simulink model "Tractor_Model"  (R2022b)
settings: Solver=daessc  StartTime=0.0  StopTime=80  FixedStep=1  MaxStep=.01  RelTol=1
libraries: nesl_utility x12, fl_lib x6, sdl_lib x5, simulink x2
settings Model: Creator=david  LastModifiedBy=david
settings SolverCC: ZeroCrossAlgorithm=Adaptive
settings SimscapeCC: SimscapeLogType=all

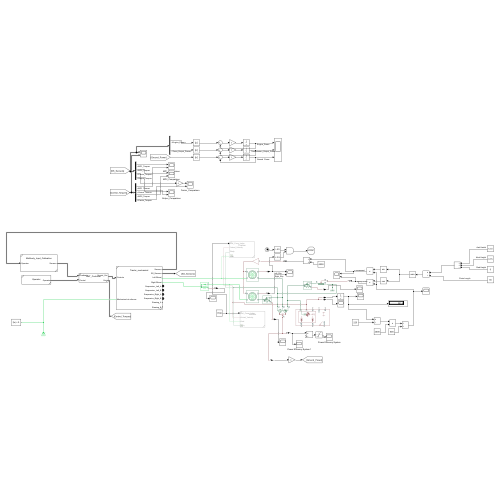
[thumbnail: Simulink's stored preview of the top-level diagram]
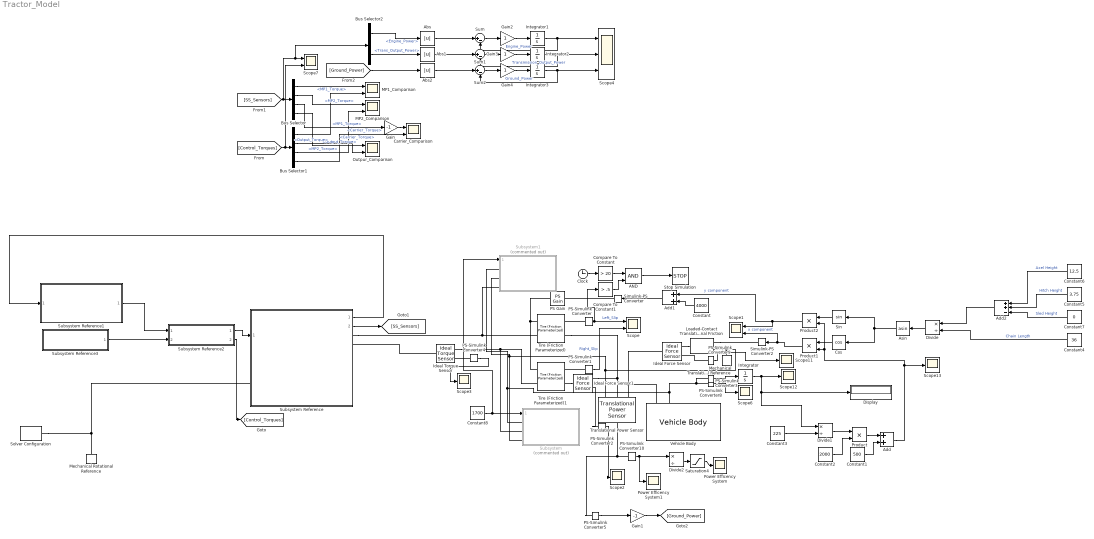
== system Tractor_Model ==
  AND : Logic  IconShape=distinctive  AllPortsSameDT=off  OutDataTypeStr=boolean
  Abs : Abs  SaturateOnIntegerOverflow=off
  Abs1 : Abs  SaturateOnIntegerOverflow=off
  Abs2 : Abs  SaturateOnIntegerOverflow=off
  Add : Sum
  Add1 : Sum
  Add2 : Sum  Inputs=++-
  Asin : Trigonometry  Operator=asin
  Bus Selector : BusSelector  OutputSignals=Trans.MP1_Torque,Trans.MP2_Torque,Trans.Carrier_Torque,Trans.Output_Torque
  Bus Selector1 : BusSelector  OutputSignals=MP1_Torque,Output_Torque,MP2_Torque,Carrier_Torque
  Bus Selector2 : BusSelector  OutputSignals=Engine_Power,Trans_Output_Power
  Carrier_Comparison : Scope  NumInputPorts=2
  Clock : Clock
  Compare To Constant : simulink/Logic and Bit Operations/Compare To Constant  relop=>  const=20  OutDataTypeStr=boolean
  Compare To Constant1 : simulink/Logic and Bit Operations/Compare To Constant  relop=>  const=.5  OutDataTypeStr=boolean
  Constant : Constant  Value=4000
  Constant1 : Constant  Value=500
  Constant2 : Constant  Value=2000
  Constant3 : Constant  Value=225
  Constant4 : Constant  Value=36
  Constant5 : Constant  Value=3.75
  Constant6 : Constant  Value=12.5
  Constant7 : Constant  Value=0
  Constant8 : Constant  Value=1700
  Cos : Trigonometry  Operator=cos
  Display : Display
  Divide : Product  Inputs=*/
  Divide1 : Product  Inputs=*/
  Divide2 : Product  Inputs=*/
  Gain : Gain  Gain=-1
  Gain1 : Gain  Gain=-1
  Gain2 : Gain
  Gain3 : Gain
  Gain4 : Gain
  Ideal Force Sensor : fl_lib/Mechanical/Mechanical Sensors/Ideal Force Sensor
  Ideal Force Sensor1 : fl_lib/Mechanical/Mechanical Sensors/Ideal Force Sensor
  Ideal Torque Sensor : fl_lib/Mechanical/Mechanical Sensors/Ideal Torque Sensor
  Integrator{,1..3} (4 alike) : Integrator
  Loaded-Contact Translational Friction : sdl_lib/Brakes & Detents/Translational/Loaded-Contact Translational Friction  friction_model=sdl.enum.friction_model_TLU_thermal.fixed  mu_v_vector=[0, .1, 1] m/s  temperature_TLU=[280, 300, 320] K  mu_static=2  mu_static_vector=[.4, .38, .36]  mu_coulomb=1  mu_coulomb_vector=[.3, .22, .19]  mu_coulomb_temp_vector=[.3, .28, .25]  mu_coulomb_matrix=[.34, .32, .3; .3, .28, .25; .25, .2, .15]  mu_interp_method=simscape.enum.interpolation.linear  mu_extrap_method=simscape.enum.extrapolation.linear  v_tol=0.001 m/s  force_min=1 N  mu_visc=0 N*s/m  initial_state_locked=sdl.enum.initial_lock.unlocked  enable_faults=simscape.enum.onoff.off  fault_type=sdl.enum.clutchFault.lock  external_fault=simscape.enum.onoff.off  temporal_fault=simscape.enum.onoff.off  fault_time=5 s  report_fault=simscape.enum.assert.action.none  thermal_mass=50 kJ/K  T_init=300 K
      settings: InternalSimscapePortConfiguration="{\"Bottom\":[],\"Left\":[{\"id\":\"N\",\"label\":\"N\",\"type\":\"input\"},{\"id\":\"B\",\"label\":\"B\",\"type\":\"foundation.mechanical.translational.translational\"}],\"Right\":[{\"id\":\"F\",\"label\":\"F\",\"type\":\"foundation.mechanical.translational.translational\"}],\"Top\":[]}"
  MP1_Comparison : Scope  NumInputPorts=2
  MP2_Comparison : Scope  NumInputPorts=2
  Mechanical Rotational Reference : fl_lib/Mechanical/Rotational Elements/Mechanical Rotational Reference
  Mechanical Translational Reference : fl_lib/Mechanical/Translational Elements/Mechanical Translational Reference
  Outpur_Comparison : Scope  NumInputPorts=2
  PS Gain : fl_lib/Physical Signals/Functions/PS Gain  gain=.5
  PS-Simulink Converter{,1..2,4} (4 alike) : nesl_utility/PS-Simulink Converter  PhysicalDomain=network_engine_domain  SubClassName=ps_output  LeftPortType=input  RightPortType=output  PseudoPeriodic=off  Frequencies=[]  VectorFormat=inherit  Unit=inherit  AffineConversion=off
  PS-Simulink Converter10 : nesl_utility/PS-Simulink Converter  PhysicalDomain=network_engine_domain  SubClassName=ps_output  LeftPortType=input  RightPortType=output  PseudoPeriodic=off  Frequencies=[]  VectorFormat=inherit  Unit=HP_DIN  AffineConversion=off
  PS-Simulink Converter3 : nesl_utility/PS-Simulink Converter  PhysicalDomain=network_engine_domain  SubClassName=ps_output  LeftPortType=input  RightPortType=output  PseudoPeriodic=off  Frequencies=[]  VectorFormat=inherit  Unit=mph  AffineConversion=off
  PS-Simulink Converter5 : nesl_utility/PS-Simulink Converter  PhysicalDomain=network_engine_domain  SubClassName=ps_output  LeftPortType=input  RightPortType=output  PseudoPeriodic=off  Frequencies=[]  VectorFormat=inherit  Unit=W  AffineConversion=off
  PS-Simulink Converter8 : nesl_utility/PS-Simulink Converter  PhysicalDomain=network_engine_domain  SubClassName=ps_output  LeftPortType=input  RightPortType=output  PseudoPeriodic=off  Frequencies=[]  VectorFormat=inherit  Unit=fps  AffineConversion=off
  PS-Simulink Converter9 : nesl_utility/PS-Simulink Converter  PhysicalDomain=network_engine_domain  SubClassName=ps_output  LeftPortType=input  RightPortType=output  PseudoPeriodic=off  Frequencies=[]  VectorFormat=inherit  Unit=lbf  AffineConversion=off
  Power Efficency System : Scope
  Power Efficency System1 : Scope
  Product : Product
  Product1 : Product
  Product2 : Product
  Saturation4 : Saturate  UpperLimit=1  LowerLimit=0
  Scope : Scope  NumInputPorts=2
  Scope1 : Scope  NumInputPorts=2
  Scope{2..3,6,11..13} (6 alike) : Scope
  Scope4 : Scope  NumInputPorts=3
  Scope7 : Scope  NumInputPorts=2
  Simulink-PS Converter : nesl_utility/Simulink-PS Converter  PhysicalDomain=network_engine_domain  SubClassName=ps_input  LeftPortType=input  RightPortType=output  PseudoPeriodic=off  Frequencies=[]  NoiseDistribution=none  NoiseParameters=[]  Unit=lbf  AffineConversion=off  FilteringAndDerivatives=provide  SimscapeFilterOrder=1  InputFilterTimeConstant=0.001  UdotUserProvided=0
  Simulink-PS Converter2 : nesl_utility/Simulink-PS Converter  PhysicalDomain=network_engine_domain  SubClassName=ps_input  LeftPortType=input  RightPortType=output  PseudoPeriodic=off  Frequencies=[]  NoiseDistribution=none  NoiseParameters=[]  Unit=lbf  AffineConversion=off  FilteringAndDerivatives=provide  SimscapeFilterOrder=1  InputFilterTimeConstant=0.001  UdotUserProvided=0
  Sin : Trigonometry
  Solver Configuration : nesl_utility/Solver Configuration  PhysicalDomain=network_engine_domain  SubClassName=solver  LeftPortType=input  RightPortType=generic  Tones=[]  Harmonics=[]  SimulateNoise=off  Profile=off  UseLocalSampling=off  EnableSwitchedLinearOptims=on  FrequencyDomain=off  UseCCode=off  RelTol=0.001  AbsTol=0.001  MinStep=1e-09  ToWorkspace=off  RevertToSquareIcSolve=off  NumHomotopyIterations=100  PhasorMode=off  PhasorModeNumHarmonics=1  ConsistencySolver=NEWTON_XTOL_AFTER_FTOL  IndexReductionMethod=DerivativeReplacement  DoDC=off  ResidualTolerance=1e-09  ConsistencyTolSource=LOCAL  ConsistencyAbsTol=0.1  ConsistencyRelTol=0.1  ConsistencyTolFactor=0.1  UseLocalSolver=on  LocalSolverChoice=NE_BACKWARD_EULER_ADVANCER  ResolveIndetEquations=on  FunctionEvalNumThread=1  LocalSolverSampleTime=0.001  DoFixedCost=on  MaxNonlinIter=3  MaxModeIter=2  ComputeImpulses=off  ImpulseIterations=2  LinearAlgebra=auto  LinearAlgebraNumThread=0  EquationFormulation=NE_TIME_EF  DelaysMemoryBudget=1024  AutomaticFiltering=on  FilteringTimeConstant=0.001  PartitionStorageMethod=AS_NEEDED  PartitionMemoryBudget=1024  PartitionMethod=ROBUST
  Stop Simulation : Stop
  Subsystem : Subsystem  Commented=on  ReferencedSubsystem=Traction
  Subsystem Reference : Subsystem  ReferencedSubsystem=Tractor_mechanical
  Subsystem Reference1 : Subsystem  ReferencedSubsystem=Multibody_Input_Calibration
  Subsystem Reference2 : Subsystem  ReferencedSubsystem=HMT_Controller
  Subsystem Reference3 : Subsystem  ReferencedSubsystem=Operator
  Subsystem1 : Subsystem  Commented=on  ReferencedSubsystem=Traction
      settings: PortSchema="{\"entries\":[{\"content\":{\"sides\":[{\"content\":{\"connectorIds\":[\"In1\",\"LConn1\",\"LConn3\",\"LConn2\"]},\"type\":\"ConnectorPlacement.EquallySpacedRectSide\",\"uuid\":\"7553e61f-24b3-4d2c-a3de-6199074152e5\"},{\"content\":{\"connectorIds\":[],\"side\":\"RIGHT\"},\"type\":\"ConnectorPlacement.EquallySpacedRectSide\",\"uuid\":\"e7ac914d-dd58-4fb5-8222-660786b0a9ec\"},{\"content\":{\"connectorIds\":[],\"side\":\"TOP\"},\"type\":\"ConnectorPlacement.EquallySpacedRectSide\",\"uuid\":\"bf959b50-4606-428f-a1d5-18d4a5d84708\"}]},\"type\":\"ConnectorPlacement.EquallySpacedConnector\",\"uuid\":\"ba497064-9a98-429f-afaa-eb697e7869a3\"}],\"packageUris\":[\"http://schema.mathworks.com/mf0/Connector/R2020b\"],\"version\":\"1.0\"}"
  Sum : Sum  Inputs=|+-
  Sum1 : Sum  Inputs=|+-
  Sum2 : Sum  Inputs=|+-
  Tire (Friction Parameterized) : sdl_lib/Tires & Vehicles/Tire (Friction Parameterized)  r_tire=26 in  slip_output=sdl.enum.SlipOutput.Relative  friction_model=sdl.enum.friction_model_var.fixed  mu_static=0.85  mu_kinetic=0.7  slip_vector=[0, .02, .06, .15, .6, 1] rad/s  mu_kinetic_vector=[.89, .88, .8, .75, .7, .7]  interp_method=simscape.enum.interpolation.linear  extrap_method=simscape.enum.extrapolation.linear  model_compliance=sdl.enum.compliance.off  stiffness=1e6 N/m  damping=1000 N*s/m  model_inertia=sdl.enum.model_inertia.off  tire_inertia=1 kg*m^2  initial_velocity=0 rad/s  model_resistance=simscape.enum.onoff.off  resistance_model=sdl.enum.rollingResistanceParameterization.constant  coeff=0.015  p_tire=250e3 Pa  alpha=-0.003  beta=0.97  coeff_a=84e-4  coeff_b=6.2e-4 s/m  coeff_c=1.6e-4 s^2/m^2  v_thr=0.001 m/s  v_tol=0.01 m/s  F_min=10 N  initial_traction_state=sdl.enum.tireIC.traction
      settings: InternalSimscapePortConfiguration="{\"Bottom\":[],\"Left\":[{\"id\":\"N\",\"label\":\"N\",\"type\":\"input\"},{\"id\":\"A\",\"label\":\"A\",\"type\":\"foundation.mechanical.rotational.rotational\"}],\"Right\":[{\"id\":\"Srel\",\"label\":\"S\",\"type\":\"output\"},{\"id\":\"H\",\"label\":\"H\",\"type\":\"foundation.mechanical.translational.translational\"}],\"Top\":[]}"
  Tire (Friction Parameterized)1 : sdl_lib/Tires & Vehicles/Tire (Friction Parameterized)  r_tire=26 in  slip_output=sdl.enum.SlipOutput.Relative  friction_model=sdl.enum.friction_model_var.fixed  mu_static=0.85  mu_kinetic=0.7  slip_vector=[0, .02, .06, .15, .6, 1] rad/s  mu_kinetic_vector=[.89, .88, .8, .75, .7, .7]  interp_method=simscape.enum.interpolation.linear  extrap_method=simscape.enum.extrapolation.linear  model_compliance=sdl.enum.compliance.off  stiffness=1e6 N/m  damping=1000 N*s/m  model_inertia=sdl.enum.model_inertia.off  tire_inertia=1 kg*m^2  initial_velocity=0 rad/s  model_resistance=simscape.enum.onoff.on  resistance_model=sdl.enum.rollingResistanceParameterization.constant  coeff=0.015  p_tire=250e3 Pa  alpha=-0.003  beta=0.97  coeff_a=84e-4  coeff_b=6.2e-4 s/m  coeff_c=1.6e-4 s^2/m^2  v_thr=0.001 m/s  v_tol=0.01 m/s  F_min=10 N  initial_traction_state=sdl.enum.tireIC.traction
      settings: InternalSimscapePortConfiguration="{\"Bottom\":[],\"Left\":[{\"id\":\"N\",\"label\":\"N\",\"type\":\"input\"},{\"id\":\"A\",\"label\":\"A\",\"type\":\"foundation.mechanical.rotational.rotational\"}],\"Right\":[{\"id\":\"Srel\",\"label\":\"S\",\"type\":\"output\"},{\"id\":\"H\",\"label\":\"H\",\"type\":\"foundation.mechanical.translational.translational\"}],\"Top\":[]}"
  Translational Power Sensor : sdl_lib/Sensors/Translational Power Sensor  measurement_type=sdl.enum.translationalPowerSensorType.instantaneous  averaging_period=1 s  max_frequency=1000 Hz
      settings: InternalSimscapePortConfiguration="{\"Bottom\":[],\"Left\":[{\"id\":\"S\",\"label\":\"S\",\"type\":\"foundation.mechanical.translational.translational\"},{\"id\":\"R\",\"label\":\"R\",\"type\":\"foundation.mechanical.translational.translational\"},{\"id\":\"C\",\"label\":\"C\",\"type\":\"foundation.mechanical.translational.translational\"}],\"Right\":[{\"id\":\"P\",\"label\":\"P\",\"type\":\"output\"}],\"Top\":[]}"
  Vehicle Body : sdl_lib/Tires & Vehicles/Vehicle Body  mass=10000 lbm  n_w=2  x_f=1.4 m  x_r=1.6 m  y_c=0.5 m  mass_var=simscape.enum.onoff.on  g=9.81 m/s^2  liftoff_warning=simscape.enum.onoff.off  area=3 m^2  Cd=0.4  rho=1.18 kg/m^3  model_pitch=simscape.enum.onoff.off  inertia=4000 kg*m^2  suspension_model=sdl.enum.linearTLU.linear  k_f=1e4 N/m  b_f=1e4 N*s/m  k_r=1e4 N/m  b_r=1e4 N*s/m  k_f_TLU=[-2000, -1000, 0, 1000, 2000] N  x_f_TLU=[-.4, -.2, 0, .2, .4] m  b_f_TLU=[-200, -100, 0, 100, 200] N  v_f_TLU=[-4, -2, 0, 2, 4] m/s  k_r_TLU=[-2000, -1000, 0, 1000, 2000] N  x_r_TLU=[-.4, -.2, 0, .2, .4] m  b_r_TLU=[-200, -100, 0, 100, 200] N  v_r_TLU=[-4, -2, 0, 2, 4] m/s  interp_method=simscape.enum.interpolation.linear  extrap_method=simscape.enum.extrapolation.linear  model_hardstop=simscape.enum.onoff.off  upper_bound_f=.25 m  lower_bound_f=-.25 m  stop_k_f=1e6 N/m  stop_b_f=150 N*s/m  upper_bound_r=.25 m  lower_bound_r=-.25 m  stop_k_r=1e6 N/m  stop_b_r=150 N*s/m  initial_pitch=0 rad  initial_pitch_rate=0 rad/s  v_specify=off  v_priority=High  v=0 m/s  v_nominal_specify=off  v_nominal_unit=m/s  v_nominal_value=1
      settings: InternalSimscapePortConfiguration="{\"Bottom\":[],\"Left\":[{\"id\":\"H\",\"label\":\"H\",\"type\":\"foundation.mechanical.translational.translational\"},{\"id\":\"V\",\"label\":\"V\",\"type\":\"output\"},{\"id\":\"wind\",\"label\":\"W\",\"type\":\"input\"},{\"id\":\"cg_load\",\"label\":\"CG\",\"type\":\"input\"},{\"id\":\"mass_load\",\"label\":\"M\",\"type\":\"input\"}],\"Right\":[{\"id\":\"NR\",\"label\":\"NR\",\"type\":\"output\"},{\"id\":\"NF\",\"label\":\"NF\",\"type\":\"output\"},{\"id\":\"beta\",\"label\":\"beta\",\"type\":\"input\"}],\"Top\":[]}"
  wires:
  PS-Simulink Converter3/1 -> Scope6/1
  PS-Simulink Converter8/1 -> Integrator/1
  Integrator/1 -> Display/1, Divide1/1, Scope12/1
  Constant3/1 -> Divide1/2
  Divide1/1 -> Product/1
  Constant2/1 -> Product/2
  Product/1 -> Add/1
  Constant1/1 -> Add/2
  Add/1 -> Product2/2, Product1/2, Scope13/1
  PS-Simulink Converter9/1 -> Scope11/1
  Saturation4/1 -> Power Efficency System/1
  Divide2/1 -> Saturation4/1
  PS-Simulink Converter10/1 -> Power Efficency System1/1, Divide2/1
  Add1/1 -> Simulink-PS Converter/1
  Constant/1 -> Add1/2
  Cos/1 -> Product1/1
  Sin/1 -> Product2/1
  Product1/1 -> Scope1/2, Simulink-PS Converter2/1  "x component"
  Product2/1 -> Scope1/1, Add1/1  "y component"
  Asin/1 -> Cos/1, Sin/1
  Constant4/1 -> Divide/2  "Chain Length"
  Divide/1 -> Asin/1
  Add2/1 -> Divide/1
  Constant5/1 -> Add2/2  "Hitch Height"
  Constant6/1 -> Add2/1  "Axel Height"
  Constant7/1 -> Add2/3  "Sled Height"
  Subsystem Reference2/1 -> Subsystem Reference/1
  Subsystem Reference1/1 -> Subsystem Reference2/1
  Subsystem Reference3/1 -> Subsystem Reference2/2
  Subsystem Reference/1 -> Subsystem Reference1/1
  Constant8/1 -> Subsystem1/1, Subsystem/1
  PS-Simulink Converter/1 -> Compare To Constant1/1, Scope/1  "Left_Slip"
  PS-Simulink Converter1/1 -> Scope/2  "Right_Slip"
  Subsystem Reference2/2 -> [Control_Torques]
  Subsystem Reference/2 -> [SS_Sensors]
  [SS_Sensors] -> Bus Selector2/1, Scope7/1, Bus Selector/1
  [Control_Torques] -> Scope7/2, Bus Selector1/1
  Bus Selector/1 -> MP1_Comparison/1  "<MP1_Torque>"
  Bus Selector1/1 -> MP1_Comparison/2  "<MP1_Torque>"
  Bus Selector/2 -> MP2_Comparison/1  "<MP2_Torque>"
  Bus Selector1/3 -> MP2_Comparison/2  "<MP2_Torque>"
  Bus Selector/3 -> Gain/1  "<Carrier_Torque>"
  Bus Selector1/4 -> Carrier_Comparison/2  "<Carrier_Torque>"
  Bus Selector/4 -> Outpur_Comparison/1  "<Output_Torque>"
  Bus Selector1/2 -> Outpur_Comparison/2  "<Output_Torque>"
  Gain/1 -> Carrier_Comparison/1
  Clock/1 -> Compare To Constant/1
  Compare To Constant/1 -> AND/1
  Compare To Constant1/1 -> AND/2
  AND/1 -> Stop Simulation/1
  PS-Simulink Converter2/1 -> Scope2/1
  PS-Simulink Converter4/1 -> Scope3/1
  Gain1/1 -> [Ground_Power]
  Bus Selector2/1 -> Abs/1  "<Engine_Power>"
  [Ground_Power] -> Abs2/1
  PS-Simulink Converter5/1 -> Gain1/1
  Bus Selector2/2 -> Abs1/1  "<Trans_Output_Power>"
  Integrator1/1 -> Sum/2, Scope4/1  "Engine_Power"
  Gain2/1 -> Integrator1/1
  Sum/1 -> Gain2/1
  Abs/1 -> Sum/1
  Abs1/1 -> Sum1/1
  Sum1/1 -> Gain3/1
  Gain3/1 -> Integrator2/1
  Integrator2/1 -> Scope4/2, Sum1/2  "Transmission_Output_Power"
  Integrator3/1 -> Scope4/3, Sum2/2  "Ground_Power"
  Gain4/1 -> Integrator3/1
  Sum2/1 -> Gain4/1
  Abs2/1 -> Sum2/1
  connections:
  PS-Simulink Converter3/LConn1 -- PS-Simulink Converter8/LConn1 -- Subsystem/LConn1 -- Subsystem1/LConn1 -- Vehicle Body/LConn2
  Loaded-Contact Translational Friction/LConn1 -- Simulink-PS Converter2/RConn1
  Mechanical Translational Reference/LConn1 -- Subsystem/LConn3 -- Subsystem1/LConn3 -- Translational Power Sensor/LConn3 -- Loaded-Contact Translational Friction/LConn2
  Ideal Force Sensor/RConn1 -- Loaded-Contact Translational Friction/RConn1
  PS-Simulink Converter9/LConn1 -- Ideal Force Sensor/RConn2
  Tire (Friction Parameterized)/RConn2 -- Ideal Force Sensor1/RConn1 -- Translational Power Sensor/LConn2
  Translational Power Sensor/LConn1 -- Vehicle Body/LConn1 -- Ideal Force Sensor/LConn1
  PS-Simulink Converter10/LConn1 -- Translational Power Sensor/RConn1 -- PS-Simulink Converter5/LConn1
  Solver Configuration/RConn1 -- Subsystem Reference/LConn1 -- Mechanical Rotational Reference/LConn1
  PS Gain/RConn1 -- Tire (Friction Parameterized)1/LConn1 -- Tire (Friction Parameterized)/LConn1
  Simulink-PS Converter/RConn1 -- PS Gain/LConn1
  Subsystem Reference/RConn1 -- Subsystem1/LConn2 -- Tire (Friction Parameterized)/LConn2
  Ideal Torque Sensor/RConn1 -- Subsystem/LConn2 -- Tire (Friction Parameterized)1/LConn2
  PS-Simulink Converter/LConn1 -- Tire (Friction Parameterized)/RConn1
  PS-Simulink Converter1/LConn1 -- Tire (Friction Parameterized)1/RConn1
  Tire (Friction Parameterized)1/RConn2 -- Ideal Force Sensor1/LConn1
  PS-Simulink Converter2/LConn1 -- Ideal Force Sensor1/RConn2
  Ideal Torque Sensor/LConn1 -- Subsystem Reference/RConn2
  PS-Simulink Converter4/LConn1 -- Ideal Torque Sensor/RConn2
